simulink subsystem "LQR_controller"  (R2022b)
settings: Solver=VariableStepAuto  StartTime=0.0  StopTime=10.0  RelTol=1e-3
model mask{Kx=0, Ke=0}
  mask prompts: Kx "Kx - State Feedback Gain:"; Ke "Ke - Error Gain:"
settings Model: Creator=gotta  LastModifiedBy=gotta

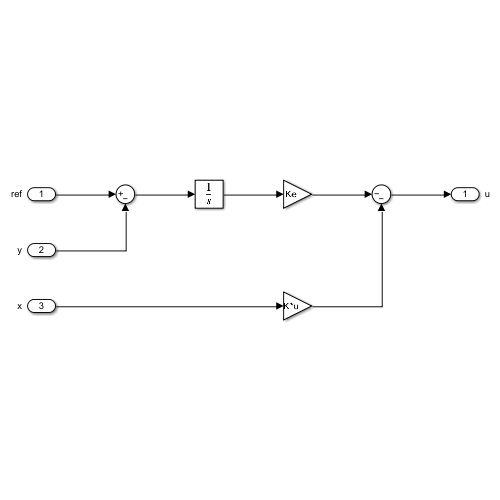
[thumbnail: Simulink's stored preview of the top-level diagram]
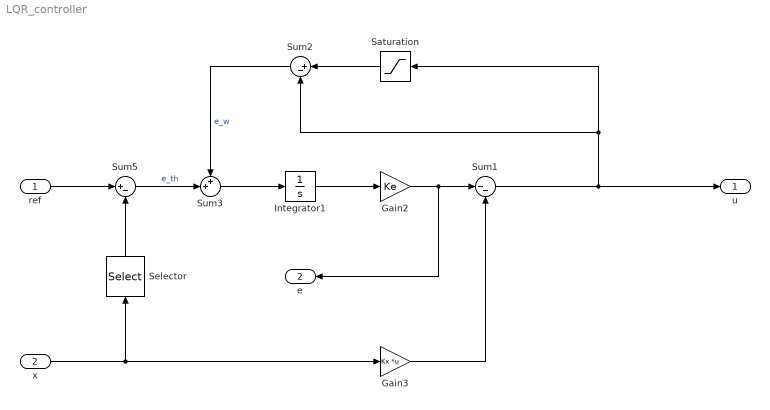
== system LQR_controller ==
  ref : Inport
  x : Inport  Port=2
  Gain2 : Gain  Gain=Ke
  Gain3 : Gain  Gain=Kx  Multiplication=Matrix(K*u)
  Integrator1 : Integrator  UpperSaturationLimit=2  LowerSaturationLimit=-2
  Saturation : Saturate  UpperLimit=1  LowerLimit=-1
  Selector : Selector  InputPortWidth=3  IndexOptions=Index vector (dialog)  Indices=1  OutputSizes=1
  Sum1 : Sum  Inputs=|--
  Sum2 : Sum  Inputs=|+-
  Sum3 : Sum  Inputs=++|
  Sum5 : Sum  Inputs=|+-
  u : Outport
  e : Outport  Port=2
  wires:
  Gain2/1 -> Sum1/1, e/1
  Saturation/1 -> Sum2/1
  Integrator1/1 -> Gain2/1
  Sum1/1 -> Sum2/2, Saturation/1, u/1
  Gain3/1 -> Sum1/2
  x/1 -> Gain3/1, Selector/1
  Sum5/1 -> Sum3/2  "e_th"
  Sum3/1 -> Integrator1/1
  Sum2/1 -> Sum3/1  "e_w"
  ref/1 -> Sum5/1
  Selector/1 -> Sum5/2
